simulink model "control_2016"  (R2016b)
settings: Solver=VariableStepAuto  StartTime=0.0  StopTime=10.0  RelTol=1e-3
settings Model: Creator=mikkelsorensen  LastModifiedBy=mikkelsorensen

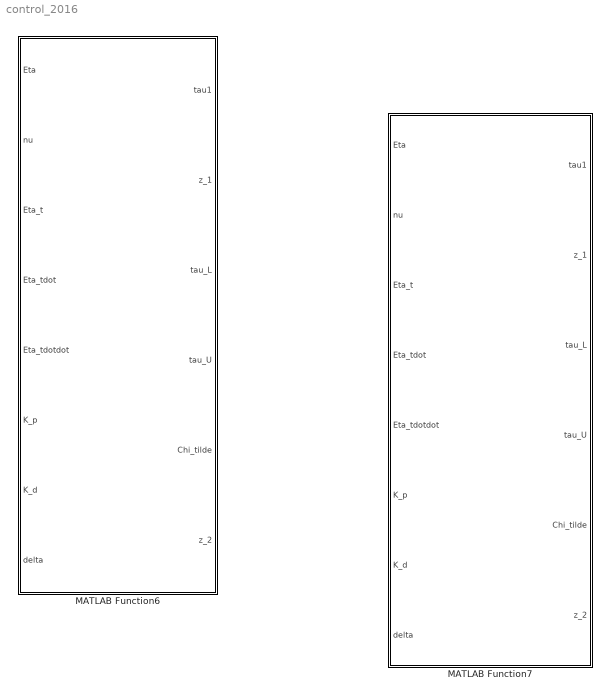
== system control_2016 ==
  MATLAB Function6 : MATLAB Function  TreatAsAtomicUnit=on
  MATLAB Function7 : MATLAB Function  TreatAsAtomicUnit=on

== matlab function control_2016/MATLAB Function6 ==
  data: Eta input; tau1 output; z_1 output; tau_L output; tau_U output; Chi_tilde output; nu input; Eta_t input; Eta_tdot input; Eta_tdotdot input; z_2 output; K_p input; K_d input; delta input
  function [ tau1,z_1,tau_L,tau_U,Chi_tilde,z_2] = Cascaded_feedback_controller_NP_LV(Eta,nu,Eta_t,Eta_tdot,Eta_tdotdot,K_p,K_d,delta)
%  [ tau,theta ] = Adaptiv_controller(Eta,nu,nu_dot,phi,theta_t,Eta_d,Eta_dtheta,Eta_dtheta2,v_s,v_stheta,v_st,h)
%UNTITLED6 Summary of this function goes here Skjetne
%   Detailed explanation goes here
%kan være den må løses på en smartere måte
%include Model_c to path
%#codegen
persistent PHI OMEGA_N EPSI_RR EPSI_PHI RR PHIPHI p_r p_p S_old_RR S_old_PHI pp YY_r YY_phi


stored_data=20;
if (isempty(PHI)||isempty(OMEGA_N))
    PHI=zeros(8,1);
    OMEGA_N=zeros(3,1);
    PHIPHI=zeros(8,3*stored_data);
    RR=zeros(3,3*stored_data);
    EPSI_RR=zeros(3*stored_data,1);
    EPSI_PHI=zeros(3*stored_data,1);
    S_old_RR=0;
    S_old_PHI=0;
    p_r=1;
    p_p=1;
    pp=1;
    YY_r=zeros(3*stored_data,1);
    YY_phi=zeros(3*stored_data,1);
end

 m    = 14.79;     x_g = 0.0375;   I_z  =  1.7600;  
 
 X_ud  =     -2.0;											% Table B.1
					Y_vd =     -10.0;	N_vd =    -0.0;		% Table B.1
					Y_rd =      -0.0;	N_rd =    -1.0;		% Table B.1

    M_RB_c=[m     0      0;
          0     m      m*x_g;
          0     m*x_g  I_z];
    M_A_c=[-X_ud    0          0;
            0          -Y_vd  -Y_rd;
            0          -N_vd  -N_rd];     
    M_c=M_RB_c+M_A_c;
    
    %   
%% Damping coefficients
% Comments at the end of the lines indicate the old values used.
X_u		= -0.6555;		X_v		= 0;
X_uu 	= 0.3545;		X_vv	= -2.443;
X_uuu 	= -3.787;		X_vvv	= 0;

						Y_v		= -1.33; 			Y_r		= -7.250; % Y_r
						Y_vv	= -2.776;			Y_rr	= -3.450; % Y_rr
						Y_vvv	= -64.91;			Y_rrr	= 0;
						
						Y_rv	= -0.805;			Y_vr	= -0.845; % Y_rv, Y_vr

						N_v		= 0;				N_r		= -1.900; % N_r
						N_vv	= -0.2088;			N_rr	= -0.750; % N_rr
						N_vvv	= 0;				N_rrr	= 0;
						
						N_rv	= 0.130;			N_vr	= 0.080; % N_rv, N_vr
    
    
    
R=Rot(Eta);

u   = nu(1);
v   = nu(2);
r   = nu(3);

d_11 = -X_u - X_uu*abs(u) - X_uuu*u^2;
d_22 = -Y_v - Y_vv*abs(v) - Y_vvv*v^2 - Y_rv*abs(r);
d_33 = -N_r - N_rr*abs(r) - N_rrr*r^2 - N_vr*abs(v); % using abs(r)

d_12 = -X_v - X_vv*v - X_vvv*v^2;
d_23 = -Y_r - Y_rr*abs(r) - Y_rrr*r^2 - Y_vr*abs(v);
d_32 = -N_v - N_vv*abs(v) - N_vvv*v^2 - N_rv*abs(r);

D    = [d_11 d_12 0
        0    d_22 d_23
        0    d_32 d_33];
  
%% controlsignaler
Eta_tilde=Eta-Eta_t;
Chi_tilde=Eta(3)-Eta_t(3);
Chi_tilde=mod(pi/2+Chi_tilde,pi)-pi/2; %%%%%%%%%%%%%%%%%%%%%%

%% New Controller
z_1=R'*(Eta_tilde);

E1 = eye(2)/sqrt([z_1(1) z_1(2)]*[z_1(1) z_1(2)]'+delta(1)^2);
E2 = 1/sqrt(z_1(3)^2+delta(2)^2);

K_1z1Delta = K_p*([E1 zeros(2,1); zeros(1,2) E2]);

Alpha_1=(-K_1z1Delta*z_1+(R')*Eta_tdot);
z_2=nu-Alpha_1;

z_1_dot=S(nu)'*z_1-K_p*z_1+z_2;
dz_1 = z_1_dot;
E3 = [z_1(1) z_1(2)]*[dz_1(1) dz_1(2)]'/([z_1(1) z_1(2)]*[z_1(1) z_1(2)]'+delta(1)^2)^(3/2)*eye(2);
E4 = z_1(3)*dz_1(3)/sqrt(z_1(3)^2+delta(2)^2);

Dot_K_1z1Delta = -K_p*([E3 zeros(2,1); zeros(1,2) E4]);


Alpha_1dot=-(Dot_K_1z1Delta*z_1+K_p*z_1_dot)+S(nu)'*R'*Eta_tdot + R'*Eta_tdotdot;

% TAU 
tau=C_c(nu)*nu+D*nu+M_c*Alpha_1dot-K_d*z_2;
tau1=tau;

%%
tau_L=-K_d*z_2+M_c*Alpha_1dot;
tau_U=C_c(nu)*nu+D*nu;

end

    function matrix=C_c(V) %%Coreolis matrix
    %#codegen
        matrix=C_RB_c(V)+C_A_c(V);
    end
      function matrix=C_RB_c(V)
      %#codegen
            m    = 14.79;     x_g = 0.0375;       % x_g  =  0.0460; % Table B.1

            u=V(1);
            v=V(2);
            r=V(3);
            matrix=[0        0       -m*(x_g*r+v);
                    0        0        m*u;
                    m*(x_g*r+v) -m*u    0]; 
      end
      function matrix=C_A_c(V)
      %#codegen
           X_ud  =     -2.0;											% Table B.1
					Y_vd =     -10.0;	N_vd =    -0.0;		% Table B.1
					Y_rd =      -0.0;		% Table B.1

            u=V(1);
            v=V(2);
            r=V(3);
        matrix=[0                                      0              Y_vd*v+0.5*(N_vd+Y_rd)*r;
               0                                       0             -X_ud*u;
               -Y_vd*v-0.5*(N_vd+Y_rd)*r         X_ud*u       0]; 
      end   
%{      
function [ d ] = G_d(nu)
      %#codegen
X_u		= -0.6555;
Y_v		= -1.33;
N_v		= 0;

    v=[nu(1) nu(2) 0]';

      D_L_uv=[-X_u    0  0 ;
            0     -Y_v 0;
            0     -N_v 0];
      d=(D_L_uv+D_NL_uv(v))*v;

end

function matrix = D_NL_uv(V)
      %#codegen


 
	
X_uu 	= 0.3545;		X_vv	= -2.443;
X_uuu 	= -3.787;	

			
Y_vv	= -2.776;			
Y_vvv	= -64.91;

N_vv	= -0.2088;	

    u=V(1);
    v=V(2);
    
     matrix=[-X_uu*abs(u)-X_uuu*u^2 0 0;
            0 -Y_vv*abs(v)-Y_vvv*v^2 0;
            0 -N_vv*abs(v) 0];
end
%}
function matrix=Rot(N)
      %#codegen

    yaw=N(3);
    matrix=[cos(yaw) -sin(yaw) 0;
            sin(yaw)  cos(yaw) 0;
            0         0        1]; 
end
%{
function R_d = Rot_dot(nu,eta)
%% takes in the nu vector 
      %#codegen


R_d=S([0 0 nu(3)])*Rot([0 0 eta(3)]);

end
%}
function [ s ] = S(r)
%UNTITLED2 Summary of this function goes here
%   Detailed explanation goes here
      %#codegen

s=[0 -r(3) r(2);
   r(3) 0 -r(1);
   -r(2) r(1) 0];

end
%{
function [ phi ] = Phi( nu )
%UNTITLED3 Summary of this function goes here
%   Detailed explanation goes here
      %#codegen

v=nu(2);
IvI=abs(v);
r=nu(3);
IrI=abs(r);

phi=[0 0 0 0 0 0 0 0;
     -IrI*v -r -IvI*r -IrI*r 0 0 0 0;
     0 0 0 0 -IrI*v -r -IvI*r -IrI*r];

end
%}

== matlab function control_2016/MATLAB Function7 ==
  data: Eta input; tau1 output; z_1 output; tau_L output; tau_U output; Chi_tilde output; nu input; Eta_t input; Eta_tdot input; Eta_tdotdot input; z_2 output; K_p input; K_d input; delta input
  function [ tau1,z_1,tau_L,tau_U,Chi_tilde,z_2] = Cascaded_feedback_controller_NP_NV(Eta,nu,Eta_t,Eta_tdot,Eta_tdotdot,K_p,K_d,delta)
%  [ tau,theta ] = Adaptiv_controller(Eta,nu,nu_dot,phi,theta_t,Eta_d,Eta_dtheta,Eta_dtheta2,v_s,v_stheta,v_st,h)
%UNTITLED6 Summary of this function goes here Skjetne
%   Detailed explanation goes here
%kan være den må løses på en smartere måte
%include Model_c to path
%#codegen
persistent PHI OMEGA_N EPSI_RR EPSI_PHI RR PHIPHI p_r p_p S_old_RR S_old_PHI pp YY_r YY_phi


stored_data=20;
if (isempty(PHI)||isempty(OMEGA_N))
    PHI=zeros(8,1);
    OMEGA_N=zeros(3,1);
    PHIPHI=zeros(8,3*stored_data);
    RR=zeros(3,3*stored_data);
    EPSI_RR=zeros(3*stored_data,1);
    EPSI_PHI=zeros(3*stored_data,1);
    S_old_RR=0;
    S_old_PHI=0;
    p_r=1;
    p_p=1;
    pp=1;
    YY_r=zeros(3*stored_data,1);
    YY_phi=zeros(3*stored_data,1);
end

 m    = 14.79;     x_g = 0.0375;   I_z  =  1.7600;  
 
 X_ud  =     -2.0;											% Table B.1
					Y_vd =     -10.0;	N_vd =    -0.0;		% Table B.1
					Y_rd =      -0.0;	N_rd =    -1.0;		% Table B.1

    M_RB_c=[m     0      0;
          0     m      m*x_g;
          0     m*x_g  I_z];
    M_A_c=[-X_ud    0          0;
            0          -Y_vd  -Y_rd;
            0          -N_vd  -N_rd];     
    M_c=M_RB_c+M_A_c;
    
    %   
%% Damping coefficients
% Comments at the end of the lines indicate the old values used.
X_u		= -0.6555;		X_v		= 0;
X_uu 	= 0.3545;		X_vv	= -2.443;
X_uuu 	= -3.787;		X_vvv	= 0;

						Y_v		= -1.33; 			Y_r		= -7.250; % Y_r
						Y_vv	= -2.776;			Y_rr	= -3.450; % Y_rr
						Y_vvv	= -64.91;			Y_rrr	= 0;
						
						Y_rv	= -0.805;			Y_vr	= -0.845; % Y_rv, Y_vr

						N_v		= 0;				N_r		= -1.900; % N_r
						N_vv	= -0.2088;			N_rr	= -0.750; % N_rr
						N_vvv	= 0;				N_rrr	= 0;
						
						N_rv	= 0.130;			N_vr	= 0.080; % N_rv, N_vr
    
    
    
R=Rot(Eta);

u   = nu(1);
v   = nu(2);
r   = nu(3);

d_11 = -X_u - X_uu*abs(u) - X_uuu*u^2;
d_22 = -Y_v - Y_vv*abs(v) - Y_vvv*v^2 - Y_rv*abs(r);
d_33 = -N_r - N_rr*abs(r) - N_rrr*r^2 - N_vr*abs(v); % using abs(r)

d_12 = -X_v - X_vv*v - X_vvv*v^2;
d_23 = -Y_r - Y_rr*abs(r) - Y_rrr*r^2 - Y_vr*abs(v);
d_32 = -N_v - N_vv*abs(v) - N_vvv*v^2 - N_rv*abs(r);

D    = [d_11 d_12 0
        0    d_22 d_23
        0    d_32 d_33];
  
%% controlsignaler
Eta_tilde=Eta-Eta_t;
Chi_tilde=Eta(3)-Eta_t(3);
Chi_tilde=mod(pi/2+Chi_tilde,pi)-pi/2; %%%%%%%%%%%%%%%%%%%%%%

%% New Controller
z_1=R'*(Eta_tilde);

E1 = eye(2)/sqrt([z_1(1) z_1(2)]*[z_1(1) z_1(2)]'+delta(1)^2);
E2 = 1/sqrt(z_1(3)^2+delta(2)^2);

K_1z1Delta = K_p*([E1 zeros(2,1); zeros(1,2) E2]);

Alpha_1=(-K_1z1Delta*z_1+(R')*Eta_tdot);
z_2=nu-Alpha_1;

z_1_dot=S(nu)'*z_1-K_p*z_1+z_2;
dz_1=z_1_dot;
E3 = [z_1(1) z_1(2)]*[dz_1(1) dz_1(2)]'/([z_1(1) z_1(2)]*[z_1(1) z_1(2)]'+delta(1)^2)^(3/2)*eye(2);
E4 = z_1(3)*dz_1(3)/sqrt(z_1(3)^2+delta(2)^2);

Dot_K_1z1Delta = -K_p*([E3 zeros(2,1); zeros(1,2) E4]);


Alpha_1dot=-(Dot_K_1z1Delta*z_1+K_p*z_1_dot)+S(nu)'*R'*Eta_tdot + R'*Eta_tdotdot;

% TAU 
tau=C_c(nu)*nu+D*nu+M_c*Alpha_1dot...
    -diag([K_d(1,1)/sqrt([z_2(1) z_2(2)]*[z_2(1) z_2(2)]'+delta(3)^2) K_d(2,2)/sqrt([z_2(1) z_2(2)]*[z_2(1) z_2(2)]'+delta(3)^2) K_d(3,3)/sqrt(z_2(3)^2+delta(4)^2)])*z_2;
tau1=tau;

%%
tau_L=-K_d*z_2+M_c*Alpha_1dot;
tau_U=C_c(nu)*nu+D*nu;

end

    function matrix=C_c(V) %%Coreolis matrix
    %#codegen
        matrix=C_RB_c(V)+C_A_c(V);
    end
      function matrix=C_RB_c(V)
      %#codegen
            m    = 14.79;     x_g = 0.0375;       % x_g  =  0.0460; % Table B.1

            u=V(1);
            v=V(2);
            r=V(3);
            matrix=[0        0       -m*(x_g*r+v);
                    0        0        m*u;
                    m*(x_g*r+v) -m*u    0]; 
      end
      function matrix=C_A_c(V)
      %#codegen
           X_ud  =     -2.0;											% Table B.1
					Y_vd =     -10.0;	N_vd =    -0.0;		% Table B.1
					Y_rd =      -0.0;		% Table B.1

            u=V(1);
            v=V(2);
            r=V(3);
        matrix=[0                                      0              Y_vd*v+0.5*(N_vd+Y_rd)*r;
               0                                       0             -X_ud*u;
               -Y_vd*v-0.5*(N_vd+Y_rd)*r         X_ud*u       0]; 
      end   
%{      
function [ d ] = G_d(nu)
      %#codegen
X_u		= -0.6555;
Y_v		= -1.33;
N_v		= 0;

    v=[nu(1) nu(2) 0]';

      D_L_uv=[-X_u    0  0 ;
            0     -Y_v 0;
            0     -N_v 0];
      d=(D_L_uv+D_NL_uv(v))*v;

end

function matrix = D_NL_uv(V)
      %#codegen


 
	
X_uu 	= 0.3545;		X_vv	= -2.443;
X_uuu 	= -3.787;	

			
Y_vv	= -2.776;			
Y_vvv	= -64.91;

N_vv	= -0.2088;	

    u=V(1);
    v=V(2);
    
     matrix=[-X_uu*abs(u)-X_uuu*u^2 0 0;
            0 -Y_vv*abs(v)-Y_vvv*v^2 0;
            0 -N_vv*abs(v) 0];
end
%}
function matrix=Rot(N)
      %#codegen

    yaw=N(3);
    matrix=[cos(yaw) -sin(yaw) 0;
            sin(yaw)  cos(yaw) 0;
            0         0        1]; 
end
%{
function R_d = Rot_dot(nu,eta)
%% takes in the nu vector 
      %#codegen


R_d=S([0 0 nu(3)])*Rot([0 0 eta(3)]);

end
%}
function [ s ] = S(r)
%UNTITLED2 Summary of this function goes here
%   Detailed explanation goes here
      %#codegen

s=[0 -r(3) r(2);
   r(3) 0 -r(1);
   -r(2) r(1) 0];

end
%{
function [ phi ] = Phi( nu )
%UNTITLED3 Summary of this function goes here
%   Detailed explanation goes here
      %#codegen

v=nu(2);
IvI=abs(v);
r=nu(3);
IrI=abs(r);

phi=[0 0 0 0 0 0 0 0;
     -IrI*v -r -IvI*r -IrI*r 0 0 0 0;
     0 0 0 0 -IrI*v -r -IvI*r -IrI*r];

end
%}
